simulink model "Control_test"  (R2014b)
settings: Solver=FixedStepDiscrete  StartTime=0.0  StopTime=Inf  FixedStep=0.001  RelTol=1e-3
PostLoadFcn:
  | , if any(exist('dsrtsu_mdlpostloadfcn', 'file') == [2, 3, 6]), try dsrtsu_mdlpostloadfcn('Execute', bdroot); catch fprintf('Error in PostLoadFcn (dsrtsu_mdlpostloadfcn) for model "%s":\n %s\n', bdroot, lasterr); end, end,
undefined symbols (not defined in the file or in its folder): dtLocal, slcm
libraries: rtican x163, simulink x14
(part 28 of 34)

== system Control_test/InputProcessing/RadarCanProcessing/Track54 ==
  Bus Creator : BusCreator  Inputs=12
  ESR_Track54 : rtican/RTICAN Receive (RX)   Reserved1=[]  Reserved2=[]  Reserved3=[]  Reserved4=[]  SfcnMessage=[]  Msg_Struct=[]  BoardTypeNo=[]  BoardNo=[]  ChannelNo=[]  Parameters=[]  DialogFcn=[]  UnitName=[]  Revision=[]  UnitValues=[]  DSProperties=struct('RTI',struct('Version',uint32(5),'BlockType',struct('isSLSource',uint8(1),'isSLSink',uint8(1),'isHWSource',uint8(0),'isHWSink',uint8(0),'isSetup',uint8(0),'isInline',uint8(1),'isNonInline',uint8(0),'isInterrupt',uint8(0),'isChannelwise',uint8(0)),'IOBoardType','RTICAN','UnitType','MESSAGE','Identifier','RX','DialogType','MSVC','BlockSet','RTICAN','SlaveProcessor','CAN'))  RTIBlockInterface=struct('OutputPortsWidth',int32([1 1 1 1 1 1 1 1 1 1 1 1]),'OutputPortsActive',[1 1 1 1 1 1 1 1 1 1 1 1],'OutputPortsName',{{'CAN_TX_TRACK_RANGE_RATE_54','CAN_TX_TRACK_MED_RANGE_MODE_54','CAN_TX_TRACK_RANGE_ACCEL_54','CAN_TX_TRACK_WIDTH_54','CAN_TX_TRACK_ROLLING_COUNT_54','CAN_TX_TRACK_BRIDGE_OBJECT_54','CAN_TX_TRACK_RANGE_54','CAN_TX_TRACK_ANGLE_54','CAN_TX_TRACK_STATUS_54','CAN_TX_TRACK_ONCOMING_54','CAN_TX_TRACK_GROUPING_CHANGED_54','CAN_TX_TRACK_LAT_RATE_54'}},'OutputPortsDataType',{{'SS_DOUBLE','SS_DOUBLE','SS_DOUBLE','SS_DOUBLE','SS_DOUBLE','SS_DOUBLE','SS_DOUBLE','SS_DOUBLE','SS_DOUBLE','SS_DOUBLE','SS_DOUBLE','SS_DOUBLE'}},'OutputPortsLabel',{{'CAN_TX_TRACK_RANGE_RATE_54','CAN_TX_TRACK_MED_RANGE_MODE_54','CAN_TX_TRACK_RANGE_ACCEL_54','CAN_TX_TRACK_WIDTH_54','CAN_TX_TRACK_ROLLING_COUNT_54','CAN_TX_TRACK_BRIDGE_OBJECT_54','CAN_TX_TRACK_RANGE_54','CAN_TX_TRACK_ANGLE_54','CAN_TX_TRACK_STATUS_54','CAN_TX_TRACK_ONCOMING_54','CAN_TX_TRACK_GROUPING_CHANGED_54','CAN_TX_TRACK_LAT_RATE_54'}},'OutputPortsLabelMode','ON','InputPortsWidth',int32(0),'InputPortsActive',0,'DialogFcn','rtican_message_interface_gui','BlockDisplay',{{'','center'}},'IconTransparency','on','ParameterTunableNames',{{}},'InitLevel',3,'BlockName',struct('Token',{{'ESR_Track54'}}),'SampleTime',{{0.01}},'TriggerPort',{{'none'}},'EnablePort',{{'none'}})  RTIBlockParameters=struct('BoardTypeNo',{{1,'OFF',[]}},'BoardNo',{{2,'ON',[1 16]}},'ChannelNo',{{2,'ON',[1 2]}},'Parameters',{{struct('DataFileSupport',struct('DataFileSelectedMaster',1,'DataFileSelectedLocal',0,'DataFileName','c:\users\mpc_car\documents\github\mpc-car\controller\dbcfiles\esr_dv3_64tgt.dbc|','DataFileDate',{{{['02-Nov-2012 20:32:52']},{['21-Mar-2013 13:39:53']},{['28-Sep-2011 17:08:52']}}},'SelectedFile',['<no file selected>'],'InterfaceFcn','rtican_dbc_file_parser'),'Options',struct('StatusSelected',0,'TimeSelected',0,'DeltaTimeSelected',0,'BytePortSelected',0,'MessageLengthSelected',0,'TriggerPort',struct('Selected',0,'TriggerType',0),'UserCoding',struct('Selected',0,'InterfaceFile','UserDecodingFile','FcnName','UserDecodeFcn','InportSelected',0,'InportWidth',1,'OutportSelected',0,'OutportWidth',1),'EnablePortSelected',0,'SignalOnPortnameSelected',1,'UseRXService',0),'Message',struct('MsgOnBlocknameSelected',1,'MsgName','ESR_Track54','MsgIdFormat',0,'MsgId',1333,'MsgLength',8,'NumSignals',12,'SampleTime',0.01,'Signal',struct('SgnName',{'CAN_TX_TRACK_RANGE_RATE_54','CAN_TX_TRACK_MED_RANGE_MODE_54','CAN_TX_TRACK_RANGE_ACCEL_54','CAN_TX_TRACK_WIDTH_54','CAN_TX_TRACK_ROLLING_COUNT_54','CAN_TX_TRACK_BRIDGE_OBJECT_54','CAN_TX_TRACK_RANGE_54','CAN_TX_TRACK_ANGLE_54','CAN_TX_TRACK_STATUS_54','CAN_TX_TRACK_ONCOMING_54','CAN_TX_TRACK_GROUPING_CHANGED_54','CAN_TX_TRACK_LAT_RATE_54'},'SgnStartBit',{0,14,16,26,30,31,32,43,53,56,57,58},'SgnLength',{14,2,10,4,1,1,11,10,3,1,1,6},'SgnType',{0,0,0,0,0,0,0,0,0,0,0,0},'ModeValue',{-1,-1,-1,-1,-1,-1,-1,-1,-1,-1,-1,-1},'DataType',{1,0,1,0,0,0,0,1,0,0,0,1},'ByteLayout',{2,2,2,2,2,2,2,2,2,2,2,2},'Factor',{0.01,1,0.05,0.5,1,1,0.1,0.1,1,1,1,0.25},'Offset',{0,0,0,0,0,0,0,0,0,0,0,0},'SgnComment',{{''},{''},{''},{''},{''},{''},{''},{''},{''},{''},{''},{''}},'SgnUnit',{'m/s','','m/s/s','m','','','m','deg','','','',''},'Min',{-81.92,0,-25.6,0,0,0,0,-51.2,0,0,0,-8},'Max',{81.91,3,25.55,7.5,1,0,204.7,51.1,7,0,0,7.75},'SLDataType',{'SS_DOUBLE','SS_DOUBLE','SS_DOUBLE','SS_DOUBLE','SS_DOUBLE','SS_DOUBLE','SS_DOUBLE','SS_DOUBLE','SS_DOUBLE','SS_DOUBLE','SS_DOUBLE','SS_DOUBLE'}),'MsgIdNumFormat',0,'MsgComment',{{''}}),'Version',1.2,'general',struct('isFromLib',0)),'OFF',[]}},'GroupId',{{struct('Group',{{'RTICAN'}},'No',4,'Behavior',{{'NAMECHANGE'}},'BlockType',{{'SINK'}},'NameChangeFlag',0),'OFF',[]}},'SFcnRTICANMessage',{{struct('MsgType','RX','SFcnPortType','Scalar','MsgName','ESR_Track54','MsgIdFormat','STD','MsgId',1333,'MsgLength',8,'NumSignals',12,'SampleTime',0.01,'Signal',struct('SgnName',{'CAN_TX_TRACK_RANGE_RATE_54','CAN_TX_TRACK_MED_RANGE_MODE_54','CAN_TX_TRACK_RANGE_ACCEL_54','CAN_TX_TRACK_WIDTH_54','CAN_TX_TRACK_ROLLING_COUNT_54','CAN_TX_TRACK_BRIDGE_OBJECT_54','CAN_TX_TRACK_RANGE_54','CAN_TX_TRACK_ANGLE_54','CAN_TX_TRACK_STATUS_54','CAN_TX_TRACK_ONCOMING_54','CAN_TX_TRACK_GROUPING_CHANGED_54','CAN_TX_TRACK_LAT_RATE_54'},'SgnStartBit',{0,14,16,26,30,31,32,43,53,56,57,58},'SgnLength',{14,2,10,4,1,1,11,10,3,1,1,6},'SgnType',{'standard','standard','standard','standard','standard','standard','standard','standard','standard','standard','standard','standard'},'ModeValue',{-1,-1,-1,-1,-1,-1,-1,-1,-1,-1,-1,-1},'DataType',{['signed int'],['unsigned int'],['signed int'],['unsigned int'],['unsigned int'],['unsigned int'],['unsigned int'],['signed int'],['unsigned int'],['unsigned int'],['unsigned int'],['signed int']},'ByteLayout',{['motorola back.'],['motorola back.'],['motorola back.'],['motorola back.'],['motorola back.'],['motorola back.'],['motorola back.'],['motorola back.'],['motorola back.'],['motorola back.'],['motorola back.'],['motorola back.']},'Factor',{0.01,1,0.05,0.5,1,1,0.1,0.1,1,1,1,0.25},'Offset',{0,0,0,0,0,0,0,0,0,0,0,0},'SLDataType',{'SS_DOUBLE','SS_DOUBLE','SS_DOUBLE','SS_DOUBLE','SS_DOUBLE','SS_DOUBLE','SS_DOUBLE','SS_DOUBLE','SS_DOUBLE','SS_DOUBLE','SS_DOUBLE','SS_DOUBLE'}),'StatusSelected','no','TimeSelected','no','DeltaTimeSelected','no','BytePortSelected','no','MessageLengthSelected','no','TriggerPort',struct('Selected','no','TriggerType',0),'UserCoding',struct('Selected','no','InterfaceFile','UserDecodingFile','FcnName','UserDecodeFcn','InportSelected','no','InportWidth',1,'OutportSelected','no','OutportWidth',1),'EnablePortSelected','no','UseRXService','no','BoardType','DS1','BoardNo',2,'ControllerNo',2),'OFF',[]}},'TLCFileName',{{'rtican_rx_message','OFF',[]}})  RTISFcnParameters=struct('SFcnRTICANMessage','struct','TLCFileName','char')  RTIBlockParaDefault=struct('BoardTypeNo',4302,'BoardNo',1,'ChannelNo',1,'Parameters',struct('DataFileSupport',struct('DataFileSelectedMaster',0,'DataFileSelectedLocal',0,'DataFileName','','DataFileDate','','SelectedFile',['<no file selected>']),'Options',struct('StatusSelected',1,'TimeSelected',1,'DeltaTimeSelected',1,'BytePortSelected',0,'MessageLengthSelected',0,'TriggerPort',struct('Selected',0,'TriggerType','rising'),'UserCoding',struct('Selected',0,'InterfaceFile','UserDecodingFile','FcnName','UserDecodeFcn','InportSelected',0,'InportWidth',1,'OutportSelected',0,'OutportWidth',1),'EnablePortSelected',0,'SignalOnPortnameSelected',1,'UseRXService',0),'Message',struct('MsgOnBlocknameSelected',0,'MsgName',['RX Message'],'MsgIdFormat',0,'MsgId',100,'MsgLength',8,'NumSignals',1,'SampleTime',-1,'Signal',struct('SgnName',['RX signal'],'SgnStartBit',0,'SgnLength',8,'SgnType',0,'ModeValue',-1,'DataType',0,'SLDataType','SS_DOUBLE','ByteLayout',0,'Factor',1,'Offset',0,'Min',0,'Max',255,'SgnComment',{{}},'SgnUnit',''),'MsgIdNumFormat',0,'MsgComment',{{''}}),'Version',1.2,'general',struct('isFromLib',1)),'GroupId',struct('Group',{{'RTICAN'}},'No',1,'Behavior',{{'NAMECHANGE'}},'BlockType',{{'SINK'}},'NameChangeFlag',0),'SFcnRTICANMessage',struct('MsgType','RX','MsgName',['RX Message'],'MsgIdFormat','STD','MsgId',100,'MsgLength',8,'NumSignals',1,'SampleTime',-1,'Signal',struct('SgnName',['RX signal'],'SgnStartBit',0,'SgnLength',8,'SgnType','standard','ModeValue',-1,'DataType',['unsigned int'],'ByteLayout',['little endian'],'SLDataType','SS_DOUBLE','Factor',1,'Offset',0),'StatusSelected','yes','TimeSelected','yes','DeltaTimeSelected','yes','BytePortSelected','no','MessageLengthSelected','no','EnablePortSelected','no','UserCoding',struct('Selected','no','InterfaceFile','UserDecodingFile','FcnName','UserDecodeFcn','InportSelected','no','InportWidth',1,'OutportSelected','no','OutportWidth',1),'TriggerPort',struct('Selected','no','TriggerType','rising'),'UseRXService','no','BoardType','DS4302','BoardNo',1,'ControllerNo',1,'SFcnPortType','Scalar'),'TLCFileName','rtican_rx_message')
      settings: AttributesFormatString=Group Id: RTICAN4\n
  Out1 : Outport
  wires:
  Bus Creator/1 -> Out1/1  "Track54"
  ESR_Track54/1 -> Bus Creator/1  "CAN_TX_TRACK_RANGE_RATE_54"
  ESR_Track54/2 -> Bus Creator/2  "CAN_TX_TRACK_MED_RANGE_MODE_54"
  ESR_Track54/3 -> Bus Creator/3  "CAN_TX_TRACK_RANGE_ACCEL_54"
  ESR_Track54/4 -> Bus Creator/4  "CAN_TX_TRACK_WIDTH_54"
  ESR_Track54/5 -> Bus Creator/5  "CAN_TX_TRACK_ROLLING_COUNT_54"
  ESR_Track54/6 -> Bus Creator/6  "CAN_TX_TRACK_BRIDGE_OBJECT_54"
  ESR_Track54/7 -> Bus Creator/7  "CAN_TX_TRACK_RANGE_54"
  ESR_Track54/8 -> Bus Creator/8  "CAN_TX_TRACK_ANGLE_54"
  ESR_Track54/9 -> Bus Creator/9  "CAN_TX_TRACK_STATUS_54"
  ESR_Track54/10 -> Bus Creator/10  "CAN_TX_TRACK_ONCOMING_54"
  ESR_Track54/11 -> Bus Creator/11  "CAN_TX_TRACK_GROUPING_CHANGED_54"
  ESR_Track54/12 -> Bus Creator/12  "CAN_TX_TRACK_LAT_RATE_54"

== system Control_test/InputProcessing/RadarCanProcessing/Track55 ==
  Bus Creator : BusCreator  Inputs=12
  ESR_Track55 : rtican/RTICAN Receive (RX)   Reserved1=[]  Reserved2=[]  Reserved3=[]  Reserved4=[]  SfcnMessage=[]  Msg_Struct=[]  BoardTypeNo=[]  BoardNo=[]  ChannelNo=[]  Parameters=[]  DialogFcn=[]  UnitName=[]  Revision=[]  UnitValues=[]  DSProperties=struct('RTI',struct('Version',uint32(5),'BlockType',struct('isSLSource',uint8(1),'isSLSink',uint8(1),'isHWSource',uint8(0),'isHWSink',uint8(0),'isSetup',uint8(0),'isInline',uint8(1),'isNonInline',uint8(0),'isInterrupt',uint8(0),'isChannelwise',uint8(0)),'IOBoardType','RTICAN','UnitType','MESSAGE','Identifier','RX','DialogType','MSVC','BlockSet','RTICAN','SlaveProcessor','CAN'))  RTIBlockInterface=struct('OutputPortsWidth',int32([1 1 1 1 1 1 1 1 1 1 1 1]),'OutputPortsActive',[1 1 1 1 1 1 1 1 1 1 1 1],'OutputPortsName',{{'CAN_TX_TRACK_RANGE_RATE_55','CAN_TX_TRACK_MED_RANGE_MODE_55','CAN_TX_TRACK_RANGE_ACCEL_55','CAN_TX_TRACK_WIDTH_55','CAN_TX_TRACK_ROLLING_COUNT_55','CAN_TX_TRACK_BRIDGE_OBJECT_55','CAN_TX_TRACK_RANGE_55','CAN_TX_TRACK_ANGLE_55','CAN_TX_TRACK_STATUS_55','CAN_TX_TRACK_ONCOMING_55','CAN_TX_TRACK_GROUPING_CHANGED_55','CAN_TX_TRACK_LAT_RATE_55'}},'OutputPortsDataType',{{'SS_DOUBLE','SS_DOUBLE','SS_DOUBLE','SS_DOUBLE','SS_DOUBLE','SS_DOUBLE','SS_DOUBLE','SS_DOUBLE','SS_DOUBLE','SS_DOUBLE','SS_DOUBLE','SS_DOUBLE'}},'OutputPortsLabel',{{'CAN_TX_TRACK_RANGE_RATE_55','CAN_TX_TRACK_MED_RANGE_MODE_55','CAN_TX_TRACK_RANGE_ACCEL_55','CAN_TX_TRACK_WIDTH_55','CAN_TX_TRACK_ROLLING_COUNT_55','CAN_TX_TRACK_BRIDGE_OBJECT_55','CAN_TX_TRACK_RANGE_55','CAN_TX_TRACK_ANGLE_55','CAN_TX_TRACK_STATUS_55','CAN_TX_TRACK_ONCOMING_55','CAN_TX_TRACK_GROUPING_CHANGED_55','CAN_TX_TRACK_LAT_RATE_55'}},'OutputPortsLabelMode','ON','InputPortsWidth',int32(0),'InputPortsActive',0,'DialogFcn','rtican_message_interface_gui','BlockDisplay',{{'','center'}},'IconTransparency','on','ParameterTunableNames',{{}},'InitLevel',3,'BlockName',struct('Token',{{'ESR_Track55'}}),'SampleTime',{{0.01}},'TriggerPort',{{'none'}},'EnablePort',{{'none'}})  RTIBlockParameters=struct('BoardTypeNo',{{1,'OFF',[]}},'BoardNo',{{2,'ON',[1 16]}},'ChannelNo',{{2,'ON',[1 2]}},'Parameters',{{struct('DataFileSupport',struct('DataFileSelectedMaster',1,'DataFileSelectedLocal',0,'DataFileName','c:\users\mpc_car\documents\github\mpc-car\controller\dbcfiles\esr_dv3_64tgt.dbc|','DataFileDate',{{{['02-Nov-2012 20:32:52']},{['21-Mar-2013 13:39:53']},{['28-Sep-2011 17:08:52']}}},'SelectedFile',['<no file selected>'],'InterfaceFcn','rtican_dbc_file_parser'),'Options',struct('StatusSelected',0,'TimeSelected',0,'DeltaTimeSelected',0,'BytePortSelected',0,'MessageLengthSelected',0,'TriggerPort',struct('Selected',0,'TriggerType',0),'UserCoding',struct('Selected',0,'InterfaceFile','UserDecodingFile','FcnName','UserDecodeFcn','InportSelected',0,'InportWidth',1,'OutportSelected',0,'OutportWidth',1),'EnablePortSelected',0,'SignalOnPortnameSelected',1,'UseRXService',0),'Message',struct('MsgOnBlocknameSelected',1,'MsgName','ESR_Track55','MsgIdFormat',0,'MsgId',1334,'MsgLength',8,'NumSignals',12,'SampleTime',0.01,'Signal',struct('SgnName',{'CAN_TX_TRACK_RANGE_RATE_55','CAN_TX_TRACK_MED_RANGE_MODE_55','CAN_TX_TRACK_RANGE_ACCEL_55','CAN_TX_TRACK_WIDTH_55','CAN_TX_TRACK_ROLLING_COUNT_55','CAN_TX_TRACK_BRIDGE_OBJECT_55','CAN_TX_TRACK_RANGE_55','CAN_TX_TRACK_ANGLE_55','CAN_TX_TRACK_STATUS_55','CAN_TX_TRACK_ONCOMING_55','CAN_TX_TRACK_GROUPING_CHANGED_55','CAN_TX_TRACK_LAT_RATE_55'},'SgnStartBit',{0,14,16,26,30,31,32,43,53,56,57,58},'SgnLength',{14,2,10,4,1,1,11,10,3,1,1,6},'SgnType',{0,0,0,0,0,0,0,0,0,0,0,0},'ModeValue',{-1,-1,-1,-1,-1,-1,-1,-1,-1,-1,-1,-1},'DataType',{1,0,1,0,0,0,0,1,0,0,0,1},'ByteLayout',{2,2,2,2,2,2,2,2,2,2,2,2},'Factor',{0.01,1,0.05,0.5,1,1,0.1,0.1,1,1,1,0.25},'Offset',{0,0,0,0,0,0,0,0,0,0,0,0},'SgnComment',{{''},{''},{''},{''},{''},{''},{''},{''},{''},{''},{''},{''}},'SgnUnit',{'m/s','','m/s/s','m','','','m','deg','','','',''},'Min',{-81.92,0,-25.6,0,0,0,0,-51.2,0,0,0,-8},'Max',{81.91,3,25.55,7.5,1,0,204.7,51.1,7,0,0,7.75},'SLDataType',{'SS_DOUBLE','SS_DOUBLE','SS_DOUBLE','SS_DOUBLE','SS_DOUBLE','SS_DOUBLE','SS_DOUBLE','SS_DOUBLE','SS_DOUBLE','SS_DOUBLE','SS_DOUBLE','SS_DOUBLE'}),'MsgIdNumFormat',0,'MsgComment',{{''}}),'Version',1.2,'general',struct('isFromLib',0)),'OFF',[]}},'GroupId',{{struct('Group',{{'RTICAN'}},'No',4,'Behavior',{{'NAMECHANGE'}},'BlockType',{{'SINK'}},'NameChangeFlag',0),'OFF',[]}},'SFcnRTICANMessage',{{struct('MsgType','RX','SFcnPortType','Scalar','MsgName','ESR_Track55','MsgIdFormat','STD','MsgId',1334,'MsgLength',8,'NumSignals',12,'SampleTime',0.01,'Signal',struct('SgnName',{'CAN_TX_TRACK_RANGE_RATE_55','CAN_TX_TRACK_MED_RANGE_MODE_55','CAN_TX_TRACK_RANGE_ACCEL_55','CAN_TX_TRACK_WIDTH_55','CAN_TX_TRACK_ROLLING_COUNT_55','CAN_TX_TRACK_BRIDGE_OBJECT_55','CAN_TX_TRACK_RANGE_55','CAN_TX_TRACK_ANGLE_55','CAN_TX_TRACK_STATUS_55','CAN_TX_TRACK_ONCOMING_55','CAN_TX_TRACK_GROUPING_CHANGED_55','CAN_TX_TRACK_LAT_RATE_55'},'SgnStartBit',{0,14,16,26,30,31,32,43,53,56,57,58},'SgnLength',{14,2,10,4,1,1,11,10,3,1,1,6},'SgnType',{'standard','standard','standard','standard','standard','standard','standard','standard','standard','standard','standard','standard'},'ModeValue',{-1,-1,-1,-1,-1,-1,-1,-1,-1,-1,-1,-1},'DataType',{['signed int'],['unsigned int'],['signed int'],['unsigned int'],['unsigned int'],['unsigned int'],['unsigned int'],['signed int'],['unsigned int'],['unsigned int'],['unsigned int'],['signed int']},'ByteLayout',{['motorola back.'],['motorola back.'],['motorola back.'],['motorola back.'],['motorola back.'],['motorola back.'],['motorola back.'],['motorola back.'],['motorola back.'],['motorola back.'],['motorola back.'],['motorola back.']},'Factor',{0.01,1,0.05,0.5,1,1,0.1,0.1,1,1,1,0.25},'Offset',{0,0,0,0,0,0,0,0,0,0,0,0},'SLDataType',{'SS_DOUBLE','SS_DOUBLE','SS_DOUBLE','SS_DOUBLE','SS_DOUBLE','SS_DOUBLE','SS_DOUBLE','SS_DOUBLE','SS_DOUBLE','SS_DOUBLE','SS_DOUBLE','SS_DOUBLE'}),'StatusSelected','no','TimeSelected','no','DeltaTimeSelected','no','BytePortSelected','no','MessageLengthSelected','no','TriggerPort',struct('Selected','no','TriggerType',0),'UserCoding',struct('Selected','no','InterfaceFile','UserDecodingFile','FcnName','UserDecodeFcn','InportSelected','no','InportWidth',1,'OutportSelected','no','OutportWidth',1),'EnablePortSelected','no','UseRXService','no','BoardType','DS1','BoardNo',2,'ControllerNo',2),'OFF',[]}},'TLCFileName',{{'rtican_rx_message','OFF',[]}})  RTISFcnParameters=struct('SFcnRTICANMessage','struct','TLCFileName','char')  RTIBlockParaDefault=struct('BoardTypeNo',4302,'BoardNo',1,'ChannelNo',1,'Parameters',struct('DataFileSupport',struct('DataFileSelectedMaster',0,'DataFileSelectedLocal',0,'DataFileName','','DataFileDate','','SelectedFile',['<no file selected>']),'Options',struct('StatusSelected',1,'TimeSelected',1,'DeltaTimeSelected',1,'BytePortSelected',0,'MessageLengthSelected',0,'TriggerPort',struct('Selected',0,'TriggerType','rising'),'UserCoding',struct('Selected',0,'InterfaceFile','UserDecodingFile','FcnName','UserDecodeFcn','InportSelected',0,'InportWidth',1,'OutportSelected',0,'OutportWidth',1),'EnablePortSelected',0,'SignalOnPortnameSelected',1,'UseRXService',0),'Message',struct('MsgOnBlocknameSelected',0,'MsgName',['RX Message'],'MsgIdFormat',0,'MsgId',100,'MsgLength',8,'NumSignals',1,'SampleTime',-1,'Signal',struct('SgnName',['RX signal'],'SgnStartBit',0,'SgnLength',8,'SgnType',0,'ModeValue',-1,'DataType',0,'SLDataType','SS_DOUBLE','ByteLayout',0,'Factor',1,'Offset',0,'Min',0,'Max',255,'SgnComment',{{}},'SgnUnit',''),'MsgIdNumFormat',0,'MsgComment',{{''}}),'Version',1.2,'general',struct('isFromLib',1)),'GroupId',struct('Group',{{'RTICAN'}},'No',1,'Behavior',{{'NAMECHANGE'}},'BlockType',{{'SINK'}},'NameChangeFlag',0),'SFcnRTICANMessage',struct('MsgType','RX','MsgName',['RX Message'],'MsgIdFormat','STD','MsgId',100,'MsgLength',8,'NumSignals',1,'SampleTime',-1,'Signal',struct('SgnName',['RX signal'],'SgnStartBit',0,'SgnLength',8,'SgnType','standard','ModeValue',-1,'DataType',['unsigned int'],'ByteLayout',['little endian'],'SLDataType','SS_DOUBLE','Factor',1,'Offset',0),'StatusSelected','yes','TimeSelected','yes','DeltaTimeSelected','yes','BytePortSelected','no','MessageLengthSelected','no','EnablePortSelected','no','UserCoding',struct('Selected','no','InterfaceFile','UserDecodingFile','FcnName','UserDecodeFcn','InportSelected','no','InportWidth',1,'OutportSelected','no','OutportWidth',1),'TriggerPort',struct('Selected','no','TriggerType','rising'),'UseRXService','no','BoardType','DS4302','BoardNo',1,'ControllerNo',1,'SFcnPortType','Scalar'),'TLCFileName','rtican_rx_message')
      settings: AttributesFormatString=Group Id: RTICAN4\n
  Out1 : Outport
  wires:
  Bus Creator/1 -> Out1/1  "Track55"
  ESR_Track55/1 -> Bus Creator/1  "CAN_TX_TRACK_RANGE_RATE_55"
  ESR_Track55/2 -> Bus Creator/2  "CAN_TX_TRACK_MED_RANGE_MODE_55"
  ESR_Track55/3 -> Bus Creator/3  "CAN_TX_TRACK_RANGE_ACCEL_55"
  ESR_Track55/4 -> Bus Creator/4  "CAN_TX_TRACK_WIDTH_55"
  ESR_Track55/5 -> Bus Creator/5  "CAN_TX_TRACK_ROLLING_COUNT_55"
  ESR_Track55/6 -> Bus Creator/6  "CAN_TX_TRACK_BRIDGE_OBJECT_55"
  ESR_Track55/7 -> Bus Creator/7  "CAN_TX_TRACK_RANGE_55"
  ESR_Track55/8 -> Bus Creator/8  "CAN_TX_TRACK_ANGLE_55"
  ESR_Track55/9 -> Bus Creator/9  "CAN_TX_TRACK_STATUS_55"
  ESR_Track55/10 -> Bus Creator/10  "CAN_TX_TRACK_ONCOMING_55"
  ESR_Track55/11 -> Bus Creator/11  "CAN_TX_TRACK_GROUPING_CHANGED_55"
  ESR_Track55/12 -> Bus Creator/12  "CAN_TX_TRACK_LAT_RATE_55"

== system Control_test/InputProcessing/RadarCanProcessing/Track56 ==
  Bus Creator : BusCreator  Inputs=12
  ESR_Track56 : rtican/RTICAN Receive (RX)   Reserved1=[]  Reserved2=[]  Reserved3=[]  Reserved4=[]  SfcnMessage=[]  Msg_Struct=[]  BoardTypeNo=[]  BoardNo=[]  ChannelNo=[]  Parameters=[]  DialogFcn=[]  UnitName=[]  Revision=[]  UnitValues=[]  DSProperties=struct('RTI',struct('Version',uint32(5),'BlockType',struct('isSLSource',uint8(1),'isSLSink',uint8(1),'isHWSource',uint8(0),'isHWSink',uint8(0),'isSetup',uint8(0),'isInline',uint8(1),'isNonInline',uint8(0),'isInterrupt',uint8(0),'isChannelwise',uint8(0)),'IOBoardType','RTICAN','UnitType','MESSAGE','Identifier','RX','DialogType','MSVC','BlockSet','RTICAN','SlaveProcessor','CAN'))  RTIBlockInterface=struct('OutputPortsWidth',int32([1 1 1 1 1 1 1 1 1 1 1 1]),'OutputPortsActive',[1 1 1 1 1 1 1 1 1 1 1 1],'OutputPortsName',{{'CAN_TX_TRACK_RANGE_RATE_56','CAN_TX_TRACK_MED_RANGE_MODE_56','CAN_TX_TRACK_RANGE_ACCEL_56','CAN_TX_TRACK_WIDTH_56','CAN_TX_TRACK_ROLLING_COUNT_56','CAN_TX_TRACK_BRIDGE_OBJECT_56','CAN_TX_TRACK_RANGE_56','CAN_TX_TRACK_ANGLE_56','CAN_TX_TRACK_STATUS_56','CAN_TX_TRACK_ONCOMING_56','CAN_TX_TRACK_GROUPING_CHANGED_56','CAN_TX_TRACK_LAT_RATE_56'}},'OutputPortsDataType',{{'SS_DOUBLE','SS_DOUBLE','SS_DOUBLE','SS_DOUBLE','SS_DOUBLE','SS_DOUBLE','SS_DOUBLE','SS_DOUBLE','SS_DOUBLE','SS_DOUBLE','SS_DOUBLE','SS_DOUBLE'}},'OutputPortsLabel',{{'CAN_TX_TRACK_RANGE_RATE_56','CAN_TX_TRACK_MED_RANGE_MODE_56','CAN_TX_TRACK_RANGE_ACCEL_56','CAN_TX_TRACK_WIDTH_56','CAN_TX_TRACK_ROLLING_COUNT_56','CAN_TX_TRACK_BRIDGE_OBJECT_56','CAN_TX_TRACK_RANGE_56','CAN_TX_TRACK_ANGLE_56','CAN_TX_TRACK_STATUS_56','CAN_TX_TRACK_ONCOMING_56','CAN_TX_TRACK_GROUPING_CHANGED_56','CAN_TX_TRACK_LAT_RATE_56'}},'OutputPortsLabelMode','ON','InputPortsWidth',int32(0),'InputPortsActive',0,'DialogFcn','rtican_message_interface_gui','BlockDisplay',{{'','center'}},'IconTransparency','on','ParameterTunableNames',{{}},'InitLevel',3,'BlockName',struct('Token',{{'ESR_Track56'}}),'SampleTime',{{0.01}},'TriggerPort',{{'none'}},'EnablePort',{{'none'}})  RTIBlockParameters=struct('BoardTypeNo',{{1,'OFF',[]}},'BoardNo',{{2,'ON',[1 16]}},'ChannelNo',{{2,'ON',[1 2]}},'Parameters',{{struct('DataFileSupport',struct('DataFileSelectedMaster',1,'DataFileSelectedLocal',0,'DataFileName','c:\users\mpc_car\documents\github\mpc-car\controller\dbcfiles\esr_dv3_64tgt.dbc|','DataFileDate',{{{['02-Nov-2012 20:32:52']},{['21-Mar-2013 13:39:53']},{['28-Sep-2011 17:08:52']}}},'SelectedFile',['<no file selected>'],'InterfaceFcn','rtican_dbc_file_parser'),'Options',struct('StatusSelected',0,'TimeSelected',0,'DeltaTimeSelected',0,'BytePortSelected',0,'MessageLengthSelected',0,'TriggerPort',struct('Selected',0,'TriggerType',0),'UserCoding',struct('Selected',0,'InterfaceFile','UserDecodingFile','FcnName','UserDecodeFcn','InportSelected',0,'InportWidth',1,'OutportSelected',0,'OutportWidth',1),'EnablePortSelected',0,'SignalOnPortnameSelected',1,'UseRXService',0),'Message',struct('MsgOnBlocknameSelected',1,'MsgName','ESR_Track56','MsgIdFormat',0,'MsgId',1335,'MsgLength',8,'NumSignals',12,'SampleTime',0.01,'Signal',struct('SgnName',{'CAN_TX_TRACK_RANGE_RATE_56','CAN_TX_TRACK_MED_RANGE_MODE_56','CAN_TX_TRACK_RANGE_ACCEL_56','CAN_TX_TRACK_WIDTH_56','CAN_TX_TRACK_ROLLING_COUNT_56','CAN_TX_TRACK_BRIDGE_OBJECT_56','CAN_TX_TRACK_RANGE_56','CAN_TX_TRACK_ANGLE_56','CAN_TX_TRACK_STATUS_56','CAN_TX_TRACK_ONCOMING_56','CAN_TX_TRACK_GROUPING_CHANGED_56','CAN_TX_TRACK_LAT_RATE_56'},'SgnStartBit',{0,14,16,26,30,31,32,43,53,56,57,58},'SgnLength',{14,2,10,4,1,1,11,10,3,1,1,6},'SgnType',{0,0,0,0,0,0,0,0,0,0,0,0},'ModeValue',{-1,-1,-1,-1,-1,-1,-1,-1,-1,-1,-1,-1},'DataType',{1,0,1,0,0,0,0,1,0,0,0,1},'ByteLayout',{2,2,2,2,2,2,2,2,2,2,2,2},'Factor',{0.01,1,0.05,0.5,1,1,0.1,0.1,1,1,1,0.25},'Offset',{0,0,0,0,0,0,0,0,0,0,0,0},'SgnComment',{{''},{''},{''},{''},{''},{''},{''},{''},{''},{''},{''},{''}},'SgnUnit',{'m/s','','m/s/s','m','','','m','deg','','','',''},'Min',{-81.92,0,-25.6,0,0,0,0,-51.2,0,0,0,-8},'Max',{81.91,3,25.55,7.5,1,0,204.7,51.1,7,0,0,7.75},'SLDataType',{'SS_DOUBLE','SS_DOUBLE','SS_DOUBLE','SS_DOUBLE','SS_DOUBLE','SS_DOUBLE','SS_DOUBLE','SS_DOUBLE','SS_DOUBLE','SS_DOUBLE','SS_DOUBLE','SS_DOUBLE'}),'MsgIdNumFormat',0,'MsgComment',{{''}}),'Version',1.2,'general',struct('isFromLib',0)),'OFF',[]}},'GroupId',{{struct('Group',{{'RTICAN'}},'No',4,'Behavior',{{'NAMECHANGE'}},'BlockType',{{'SINK'}},'NameChangeFlag',0),'OFF',[]}},'SFcnRTICANMessage',{{struct('MsgType','RX','SFcnPortType','Scalar','MsgName','ESR_Track56','MsgIdFormat','STD','MsgId',1335,'MsgLength',8,'NumSignals',12,'SampleTime',0.01,'Signal',struct('SgnName',{'CAN_TX_TRACK_RANGE_RATE_56','CAN_TX_TRACK_MED_RANGE_MODE_56','CAN_TX_TRACK_RANGE_ACCEL_56','CAN_TX_TRACK_WIDTH_56','CAN_TX_TRACK_ROLLING_COUNT_56','CAN_TX_TRACK_BRIDGE_OBJECT_56','CAN_TX_TRACK_RANGE_56','CAN_TX_TRACK_ANGLE_56','CAN_TX_TRACK_STATUS_56','CAN_TX_TRACK_ONCOMING_56','CAN_TX_TRACK_GROUPING_CHANGED_56','CAN_TX_TRACK_LAT_RATE_56'},'SgnStartBit',{0,14,16,26,30,31,32,43,53,56,57,58},'SgnLength',{14,2,10,4,1,1,11,10,3,1,1,6},'SgnType',{'standard','standard','standard','standard','standard','standard','standard','standard','standard','standard','standard','standard'},'ModeValue',{-1,-1,-1,-1,-1,-1,-1,-1,-1,-1,-1,-1},'DataType',{['signed int'],['unsigned int'],['signed int'],['unsigned int'],['unsigned int'],['unsigned int'],['unsigned int'],['signed int'],['unsigned int'],['unsigned int'],['unsigned int'],['signed int']},'ByteLayout',{['motorola back.'],['motorola back.'],['motorola back.'],['motorola back.'],['motorola back.'],['motorola back.'],['motorola back.'],['motorola back.'],['motorola back.'],['motorola back.'],['motorola back.'],['motorola back.']},'Factor',{0.01,1,0.05,0.5,1,1,0.1,0.1,1,1,1,0.25},'Offset',{0,0,0,0,0,0,0,0,0,0,0,0},'SLDataType',{'SS_DOUBLE','SS_DOUBLE','SS_DOUBLE','SS_DOUBLE','SS_DOUBLE','SS_DOUBLE','SS_DOUBLE','SS_DOUBLE','SS_DOUBLE','SS_DOUBLE','SS_DOUBLE','SS_DOUBLE'}),'StatusSelected','no','TimeSelected','no','DeltaTimeSelected','no','BytePortSelected','no','MessageLengthSelected','no','TriggerPort',struct('Selected','no','TriggerType',0),'UserCoding',struct('Selected','no','InterfaceFile','UserDecodingFile','FcnName','UserDecodeFcn','InportSelected','no','InportWidth',1,'OutportSelected','no','OutportWidth',1),'EnablePortSelected','no','UseRXService','no','BoardType','DS1','BoardNo',2,'ControllerNo',2),'OFF',[]}},'TLCFileName',{{'rtican_rx_message','OFF',[]}})  RTISFcnParameters=struct('SFcnRTICANMessage','struct','TLCFileName','char')  RTIBlockParaDefault=struct('BoardTypeNo',4302,'BoardNo',1,'ChannelNo',1,'Parameters',struct('DataFileSupport',struct('DataFileSelectedMaster',0,'DataFileSelectedLocal',0,'DataFileName','','DataFileDate','','SelectedFile',['<no file selected>']),'Options',struct('StatusSelected',1,'TimeSelected',1,'DeltaTimeSelected',1,'BytePortSelected',0,'MessageLengthSelected',0,'TriggerPort',struct('Selected',0,'TriggerType','rising'),'UserCoding',struct('Selected',0,'InterfaceFile','UserDecodingFile','FcnName','UserDecodeFcn','InportSelected',0,'InportWidth',1,'OutportSelected',0,'OutportWidth',1),'EnablePortSelected',0,'SignalOnPortnameSelected',1,'UseRXService',0),'Message',struct('MsgOnBlocknameSelected',0,'MsgName',['RX Message'],'MsgIdFormat',0,'MsgId',100,'MsgLength',8,'NumSignals',1,'SampleTime',-1,'Signal',struct('SgnName',['RX signal'],'SgnStartBit',0,'SgnLength',8,'SgnType',0,'ModeValue',-1,'DataType',0,'SLDataType','SS_DOUBLE','ByteLayout',0,'Factor',1,'Offset',0,'Min',0,'Max',255,'SgnComment',{{}},'SgnUnit',''),'MsgIdNumFormat',0,'MsgComment',{{''}}),'Version',1.2,'general',struct('isFromLib',1)),'GroupId',struct('Group',{{'RTICAN'}},'No',1,'Behavior',{{'NAMECHANGE'}},'BlockType',{{'SINK'}},'NameChangeFlag',0),'SFcnRTICANMessage',struct('MsgType','RX','MsgName',['RX Message'],'MsgIdFormat','STD','MsgId',100,'MsgLength',8,'NumSignals',1,'SampleTime',-1,'Signal',struct('SgnName',['RX signal'],'SgnStartBit',0,'SgnLength',8,'SgnType','standard','ModeValue',-1,'DataType',['unsigned int'],'ByteLayout',['little endian'],'SLDataType','SS_DOUBLE','Factor',1,'Offset',0),'StatusSelected','yes','TimeSelected','yes','DeltaTimeSelected','yes','BytePortSelected','no','MessageLengthSelected','no','EnablePortSelected','no','UserCoding',struct('Selected','no','InterfaceFile','UserDecodingFile','FcnName','UserDecodeFcn','InportSelected','no','InportWidth',1,'OutportSelected','no','OutportWidth',1),'TriggerPort',struct('Selected','no','TriggerType','rising'),'UseRXService','no','BoardType','DS4302','BoardNo',1,'ControllerNo',1,'SFcnPortType','Scalar'),'TLCFileName','rtican_rx_message')
      settings: AttributesFormatString=Group Id: RTICAN4\n
  Out1 : Outport
  wires:
  Bus Creator/1 -> Out1/1  "Track56"
  ESR_Track56/1 -> Bus Creator/1  "CAN_TX_TRACK_RANGE_RATE_56"
  ESR_Track56/2 -> Bus Creator/2  "CAN_TX_TRACK_MED_RANGE_MODE_56"
  ESR_Track56/3 -> Bus Creator/3  "CAN_TX_TRACK_RANGE_ACCEL_56"
  ESR_Track56/4 -> Bus Creator/4  "CAN_TX_TRACK_WIDTH_56"
  ESR_Track56/5 -> Bus Creator/5  "CAN_TX_TRACK_ROLLING_COUNT_56"
  ESR_Track56/6 -> Bus Creator/6  "CAN_TX_TRACK_BRIDGE_OBJECT_56"
  ESR_Track56/7 -> Bus Creator/7  "CAN_TX_TRACK_RANGE_56"
  ESR_Track56/8 -> Bus Creator/8  "CAN_TX_TRACK_ANGLE_56"
  ESR_Track56/9 -> Bus Creator/9  "CAN_TX_TRACK_STATUS_56"
  ESR_Track56/10 -> Bus Creator/10  "CAN_TX_TRACK_ONCOMING_56"
  ESR_Track56/11 -> Bus Creator/11  "CAN_TX_TRACK_GROUPING_CHANGED_56"
  ESR_Track56/12 -> Bus Creator/12  "CAN_TX_TRACK_LAT_RATE_56"

== system Control_test/InputProcessing/RadarCanProcessing/Track57 ==
  Bus Creator : BusCreator  Inputs=12
  ESR_Track57 : rtican/RTICAN Receive (RX)   Reserved1=[]  Reserved2=[]  Reserved3=[]  Reserved4=[]  SfcnMessage=[]  Msg_Struct=[]  BoardTypeNo=[]  BoardNo=[]  ChannelNo=[]  Parameters=[]  DialogFcn=[]  UnitName=[]  Revision=[]  UnitValues=[]  DSProperties=struct('RTI',struct('Version',uint32(5),'BlockType',struct('isSLSource',uint8(1),'isSLSink',uint8(1),'isHWSource',uint8(0),'isHWSink',uint8(0),'isSetup',uint8(0),'isInline',uint8(1),'isNonInline',uint8(0),'isInterrupt',uint8(0),'isChannelwise',uint8(0)),'IOBoardType','RTICAN','UnitType','MESSAGE','Identifier','RX','DialogType','MSVC','BlockSet','RTICAN','SlaveProcessor','CAN'))  RTIBlockInterface=struct('OutputPortsWidth',int32([1 1 1 1 1 1 1 1 1 1 1 1]),'OutputPortsActive',[1 1 1 1 1 1 1 1 1 1 1 1],'OutputPortsName',{{'CAN_TX_TRACK_RANGE_RATE_57','CAN_TX_TRACK_MED_RANGE_MODE_57','CAN_TX_TRACK_RANGE_ACCEL_57','CAN_TX_TRACK_WIDTH_57','CAN_TX_TRACK_ROLLING_COUNT_57','CAN_TX_TRACK_BRIDGE_OBJECT_57','CAN_TX_TRACK_RANGE_57','CAN_TX_TRACK_ANGLE_57','CAN_TX_TRACK_STATUS_57','CAN_TX_TRACK_ONCOMING_57','CAN_TX_TRACK_GROUPING_CHANGED_57','CAN_TX_TRACK_LAT_RATE_57'}},'OutputPortsDataType',{{'SS_DOUBLE','SS_DOUBLE','SS_DOUBLE','SS_DOUBLE','SS_DOUBLE','SS_DOUBLE','SS_DOUBLE','SS_DOUBLE','SS_DOUBLE','SS_DOUBLE','SS_DOUBLE','SS_DOUBLE'}},'OutputPortsLabel',{{'CAN_TX_TRACK_RANGE_RATE_57','CAN_TX_TRACK_MED_RANGE_MODE_57','CAN_TX_TRACK_RANGE_ACCEL_57','CAN_TX_TRACK_WIDTH_57','CAN_TX_TRACK_ROLLING_COUNT_57','CAN_TX_TRACK_BRIDGE_OBJECT_57','CAN_TX_TRACK_RANGE_57','CAN_TX_TRACK_ANGLE_57','CAN_TX_TRACK_STATUS_57','CAN_TX_TRACK_ONCOMING_57','CAN_TX_TRACK_GROUPING_CHANGED_57','CAN_TX_TRACK_LAT_RATE_57'}},'OutputPortsLabelMode','ON','InputPortsWidth',int32(0),'InputPortsActive',0,'DialogFcn','rtican_message_interface_gui','BlockDisplay',{{'','center'}},'IconTransparency','on','ParameterTunableNames',{{}},'InitLevel',3,'BlockName',struct('Token',{{'ESR_Track57'}}),'SampleTime',{{0.01}},'TriggerPort',{{'none'}},'EnablePort',{{'none'}})  RTIBlockParameters=struct('BoardTypeNo',{{1,'OFF',[]}},'BoardNo',{{2,'ON',[1 16]}},'ChannelNo',{{2,'ON',[1 2]}},'Parameters',{{struct('DataFileSupport',struct('DataFileSelectedMaster',1,'DataFileSelectedLocal',0,'DataFileName','c:\users\mpc_car\documents\github\mpc-car\controller\dbcfiles\esr_dv3_64tgt.dbc|','DataFileDate',{{{['02-Nov-2012 20:32:52']},{['21-Mar-2013 13:39:53']},{['28-Sep-2011 17:08:52']}}},'SelectedFile',['<no file selected>'],'InterfaceFcn','rtican_dbc_file_parser'),'Options',struct('StatusSelected',0,'TimeSelected',0,'DeltaTimeSelected',0,'BytePortSelected',0,'MessageLengthSelected',0,'TriggerPort',struct('Selected',0,'TriggerType',0),'UserCoding',struct('Selected',0,'InterfaceFile','UserDecodingFile','FcnName','UserDecodeFcn','InportSelected',0,'InportWidth',1,'OutportSelected',0,'OutportWidth',1),'EnablePortSelected',0,'SignalOnPortnameSelected',1,'UseRXService',0),'Message',struct('MsgOnBlocknameSelected',1,'MsgName','ESR_Track57','MsgIdFormat',0,'MsgId',1336,'MsgLength',8,'NumSignals',12,'SampleTime',0.01,'Signal',struct('SgnName',{'CAN_TX_TRACK_RANGE_RATE_57','CAN_TX_TRACK_MED_RANGE_MODE_57','CAN_TX_TRACK_RANGE_ACCEL_57','CAN_TX_TRACK_WIDTH_57','CAN_TX_TRACK_ROLLING_COUNT_57','CAN_TX_TRACK_BRIDGE_OBJECT_57','CAN_TX_TRACK_RANGE_57','CAN_TX_TRACK_ANGLE_57','CAN_TX_TRACK_STATUS_57','CAN_TX_TRACK_ONCOMING_57','CAN_TX_TRACK_GROUPING_CHANGED_57','CAN_TX_TRACK_LAT_RATE_57'},'SgnStartBit',{0,14,16,26,30,31,32,43,53,56,57,58},'SgnLength',{14,2,10,4,1,1,11,10,3,1,1,6},'SgnType',{0,0,0,0,0,0,0,0,0,0,0,0},'ModeValue',{-1,-1,-1,-1,-1,-1,-1,-1,-1,-1,-1,-1},'DataType',{1,0,1,0,0,0,0,1,0,0,0,1},'ByteLayout',{2,2,2,2,2,2,2,2,2,2,2,2},'Factor',{0.01,1,0.05,0.5,1,1,0.1,0.1,1,1,1,0.25},'Offset',{0,0,0,0,0,0,0,0,0,0,0,0},'SgnComment',{{''},{''},{''},{''},{''},{''},{''},{''},{''},{''},{''},{''}},'SgnUnit',{'m/s','','m/s/s','m','','','m','deg','','','',''},'Min',{-81.92,0,-25.6,0,0,0,0,-51.2,0,0,0,-8},'Max',{81.91,3,25.55,7.5,1,0,204.7,51.1,7,0,0,7.75},'SLDataType',{'SS_DOUBLE','SS_DOUBLE','SS_DOUBLE','SS_DOUBLE','SS_DOUBLE','SS_DOUBLE','SS_DOUBLE','SS_DOUBLE','SS_DOUBLE','SS_DOUBLE','SS_DOUBLE','SS_DOUBLE'}),'MsgIdNumFormat',0,'MsgComment',{{''}}),'Version',1.2,'general',struct('isFromLib',0)),'OFF',[]}},'GroupId',{{struct('Group',{{'RTICAN'}},'No',4,'Behavior',{{'NAMECHANGE'}},'BlockType',{{'SINK'}},'NameChangeFlag',0),'OFF',[]}},'SFcnRTICANMessage',{{struct('MsgType','RX','SFcnPortType','Scalar','MsgName','ESR_Track57','MsgIdFormat','STD','MsgId',1336,'MsgLength',8,'NumSignals',12,'SampleTime',0.01,'Signal',struct('SgnName',{'CAN_TX_TRACK_RANGE_RATE_57','CAN_TX_TRACK_MED_RANGE_MODE_57','CAN_TX_TRACK_RANGE_ACCEL_57','CAN_TX_TRACK_WIDTH_57','CAN_TX_TRACK_ROLLING_COUNT_57','CAN_TX_TRACK_BRIDGE_OBJECT_57','CAN_TX_TRACK_RANGE_57','CAN_TX_TRACK_ANGLE_57','CAN_TX_TRACK_STATUS_57','CAN_TX_TRACK_ONCOMING_57','CAN_TX_TRACK_GROUPING_CHANGED_57','CAN_TX_TRACK_LAT_RATE_57'},'SgnStartBit',{0,14,16,26,30,31,32,43,53,56,57,58},'SgnLength',{14,2,10,4,1,1,11,10,3,1,1,6},'SgnType',{'standard','standard','standard','standard','standard','standard','standard','standard','standard','standard','standard','standard'},'ModeValue',{-1,-1,-1,-1,-1,-1,-1,-1,-1,-1,-1,-1},'DataType',{['signed int'],['unsigned int'],['signed int'],['unsigned int'],['unsigned int'],['unsigned int'],['unsigned int'],['signed int'],['unsigned int'],['unsigned int'],['unsigned int'],['signed int']},'ByteLayout',{['motorola back.'],['motorola back.'],['motorola back.'],['motorola back.'],['motorola back.'],['motorola back.'],['motorola back.'],['motorola back.'],['motorola back.'],['motorola back.'],['motorola back.'],['motorola back.']},'Factor',{0.01,1,0.05,0.5,1,1,0.1,0.1,1,1,1,0.25},'Offset',{0,0,0,0,0,0,0,0,0,0,0,0},'SLDataType',{'SS_DOUBLE','SS_DOUBLE','SS_DOUBLE','SS_DOUBLE','SS_DOUBLE','SS_DOUBLE','SS_DOUBLE','SS_DOUBLE','SS_DOUBLE','SS_DOUBLE','SS_DOUBLE','SS_DOUBLE'}),'StatusSelected','no','TimeSelected','no','DeltaTimeSelected','no','BytePortSelected','no','MessageLengthSelected','no','TriggerPort',struct('Selected','no','TriggerType',0),'UserCoding',struct('Selected','no','InterfaceFile','UserDecodingFile','FcnName','UserDecodeFcn','InportSelected','no','InportWidth',1,'OutportSelected','no','OutportWidth',1),'EnablePortSelected','no','UseRXService','no','BoardType','DS1','BoardNo',2,'ControllerNo',2),'OFF',[]}},'TLCFileName',{{'rtican_rx_message','OFF',[]}})  RTISFcnParameters=struct('SFcnRTICANMessage','struct','TLCFileName','char')  RTIBlockParaDefault=struct('BoardTypeNo',4302,'BoardNo',1,'ChannelNo',1,'Parameters',struct('DataFileSupport',struct('DataFileSelectedMaster',0,'DataFileSelectedLocal',0,'DataFileName','','DataFileDate','','SelectedFile',['<no file selected>']),'Options',struct('StatusSelected',1,'TimeSelected',1,'DeltaTimeSelected',1,'BytePortSelected',0,'MessageLengthSelected',0,'TriggerPort',struct('Selected',0,'TriggerType','rising'),'UserCoding',struct('Selected',0,'InterfaceFile','UserDecodingFile','FcnName','UserDecodeFcn','InportSelected',0,'InportWidth',1,'OutportSelected',0,'OutportWidth',1),'EnablePortSelected',0,'SignalOnPortnameSelected',1,'UseRXService',0),'Message',struct('MsgOnBlocknameSelected',0,'MsgName',['RX Message'],'MsgIdFormat',0,'MsgId',100,'MsgLength',8,'NumSignals',1,'SampleTime',-1,'Signal',struct('SgnName',['RX signal'],'SgnStartBit',0,'SgnLength',8,'SgnType',0,'ModeValue',-1,'DataType',0,'SLDataType','SS_DOUBLE','ByteLayout',0,'Factor',1,'Offset',0,'Min',0,'Max',255,'SgnComment',{{}},'SgnUnit',''),'MsgIdNumFormat',0,'MsgComment',{{''}}),'Version',1.2,'general',struct('isFromLib',1)),'GroupId',struct('Group',{{'RTICAN'}},'No',1,'Behavior',{{'NAMECHANGE'}},'BlockType',{{'SINK'}},'NameChangeFlag',0),'SFcnRTICANMessage',struct('MsgType','RX','MsgName',['RX Message'],'MsgIdFormat','STD','MsgId',100,'MsgLength',8,'NumSignals',1,'SampleTime',-1,'Signal',struct('SgnName',['RX signal'],'SgnStartBit',0,'SgnLength',8,'SgnType','standard','ModeValue',-1,'DataType',['unsigned int'],'ByteLayout',['little endian'],'SLDataType','SS_DOUBLE','Factor',1,'Offset',0),'StatusSelected','yes','TimeSelected','yes','DeltaTimeSelected','yes','BytePortSelected','no','MessageLengthSelected','no','EnablePortSelected','no','UserCoding',struct('Selected','no','InterfaceFile','UserDecodingFile','FcnName','UserDecodeFcn','InportSelected','no','InportWidth',1,'OutportSelected','no','OutportWidth',1),'TriggerPort',struct('Selected','no','TriggerType','rising'),'UseRXService','no','BoardType','DS4302','BoardNo',1,'ControllerNo',1,'SFcnPortType','Scalar'),'TLCFileName','rtican_rx_message')
      settings: AttributesFormatString=Group Id: RTICAN4\n
  Out1 : Outport
  wires:
  Bus Creator/1 -> Out1/1  "Track57"
  ESR_Track57/1 -> Bus Creator/1  "CAN_TX_TRACK_RANGE_RATE_57"
  ESR_Track57/2 -> Bus Creator/2  "CAN_TX_TRACK_MED_RANGE_MODE_57"
  ESR_Track57/3 -> Bus Creator/3  "CAN_TX_TRACK_RANGE_ACCEL_57"
  ESR_Track57/4 -> Bus Creator/4  "CAN_TX_TRACK_WIDTH_57"
  ESR_Track57/5 -> Bus Creator/5  "CAN_TX_TRACK_ROLLING_COUNT_57"
  ESR_Track57/6 -> Bus Creator/6  "CAN_TX_TRACK_BRIDGE_OBJECT_57"
  ESR_Track57/7 -> Bus Creator/7  "CAN_TX_TRACK_RANGE_57"
  ESR_Track57/8 -> Bus Creator/8  "CAN_TX_TRACK_ANGLE_57"
  ESR_Track57/9 -> Bus Creator/9  "CAN_TX_TRACK_STATUS_57"
  ESR_Track57/10 -> Bus Creator/10  "CAN_TX_TRACK_ONCOMING_57"
  ESR_Track57/11 -> Bus Creator/11  "CAN_TX_TRACK_GROUPING_CHANGED_57"
  ESR_Track57/12 -> Bus Creator/12  "CAN_TX_TRACK_LAT_RATE_57"

== system Control_test/InputProcessing/RadarCanProcessing/Track58 ==
  Bus Creator : BusCreator  Inputs=12
  ESR_Track58 : rtican/RTICAN Receive (RX)   Reserved1=[]  Reserved2=[]  Reserved3=[]  Reserved4=[]  SfcnMessage=[]  Msg_Struct=[]  BoardTypeNo=[]  BoardNo=[]  ChannelNo=[]  Parameters=[]  DialogFcn=[]  UnitName=[]  Revision=[]  UnitValues=[]  DSProperties=struct('RTI',struct('Version',uint32(5),'BlockType',struct('isSLSource',uint8(1),'isSLSink',uint8(1),'isHWSource',uint8(0),'isHWSink',uint8(0),'isSetup',uint8(0),'isInline',uint8(1),'isNonInline',uint8(0),'isInterrupt',uint8(0),'isChannelwise',uint8(0)),'IOBoardType','RTICAN','UnitType','MESSAGE','Identifier','RX','DialogType','MSVC','BlockSet','RTICAN','SlaveProcessor','CAN'))  RTIBlockInterface=struct('OutputPortsWidth',int32([1 1 1 1 1 1 1 1 1 1 1 1]),'OutputPortsActive',[1 1 1 1 1 1 1 1 1 1 1 1],'OutputPortsName',{{'CAN_TX_TRACK_RANGE_RATE_58','CAN_TX_TRACK_MED_RANGE_MODE_58','CAN_TX_TRACK_RANGE_ACCEL_58','CAN_TX_TRACK_WIDTH_58','CAN_TX_TRACK_ROLLING_COUNT_58','CAN_TX_TRACK_BRIDGE_OBJECT_58','CAN_TX_TRACK_RANGE_58','CAN_TX_TRACK_ANGLE_58','CAN_TX_TRACK_STATUS_58','CAN_TX_TRACK_ONCOMING_58','CAN_TX_TRACK_GROUPING_CHANGED_58','CAN_TX_TRACK_LAT_RATE_58'}},'OutputPortsDataType',{{'SS_DOUBLE','SS_DOUBLE','SS_DOUBLE','SS_DOUBLE','SS_DOUBLE','SS_DOUBLE','SS_DOUBLE','SS_DOUBLE','SS_DOUBLE','SS_DOUBLE','SS_DOUBLE','SS_DOUBLE'}},'OutputPortsLabel',{{'CAN_TX_TRACK_RANGE_RATE_58','CAN_TX_TRACK_MED_RANGE_MODE_58','CAN_TX_TRACK_RANGE_ACCEL_58','CAN_TX_TRACK_WIDTH_58','CAN_TX_TRACK_ROLLING_COUNT_58','CAN_TX_TRACK_BRIDGE_OBJECT_58','CAN_TX_TRACK_RANGE_58','CAN_TX_TRACK_ANGLE_58','CAN_TX_TRACK_STATUS_58','CAN_TX_TRACK_ONCOMING_58','CAN_TX_TRACK_GROUPING_CHANGED_58','CAN_TX_TRACK_LAT_RATE_58'}},'OutputPortsLabelMode','ON','InputPortsWidth',int32(0),'InputPortsActive',0,'DialogFcn','rtican_message_interface_gui','BlockDisplay',{{'','center'}},'IconTransparency','on','ParameterTunableNames',{{}},'InitLevel',3,'BlockName',struct('Token',{{'ESR_Track58'}}),'SampleTime',{{0.01}},'TriggerPort',{{'none'}},'EnablePort',{{'none'}})  RTIBlockParameters=struct('BoardTypeNo',{{1,'OFF',[]}},'BoardNo',{{2,'ON',[1 16]}},'ChannelNo',{{2,'ON',[1 2]}},'Parameters',{{struct('DataFileSupport',struct('DataFileSelectedMaster',1,'DataFileSelectedLocal',0,'DataFileName','c:\users\mpc_car\documents\github\mpc-car\controller\dbcfiles\esr_dv3_64tgt.dbc|','DataFileDate',{{{['02-Nov-2012 20:32:52']},{['21-Mar-2013 13:39:53']},{['28-Sep-2011 17:08:52']}}},'SelectedFile',['<no file selected>'],'InterfaceFcn','rtican_dbc_file_parser'),'Options',struct('StatusSelected',0,'TimeSelected',0,'DeltaTimeSelected',0,'BytePortSelected',0,'MessageLengthSelected',0,'TriggerPort',struct('Selected',0,'TriggerType',0),'UserCoding',struct('Selected',0,'InterfaceFile','UserDecodingFile','FcnName','UserDecodeFcn','InportSelected',0,'InportWidth',1,'OutportSelected',0,'OutportWidth',1),'EnablePortSelected',0,'SignalOnPortnameSelected',1,'UseRXService',0),'Message',struct('MsgOnBlocknameSelected',1,'MsgName','ESR_Track58','MsgIdFormat',0,'MsgId',1337,'MsgLength',8,'NumSignals',12,'SampleTime',0.01,'Signal',struct('SgnName',{'CAN_TX_TRACK_RANGE_RATE_58','CAN_TX_TRACK_MED_RANGE_MODE_58','CAN_TX_TRACK_RANGE_ACCEL_58','CAN_TX_TRACK_WIDTH_58','CAN_TX_TRACK_ROLLING_COUNT_58','CAN_TX_TRACK_BRIDGE_OBJECT_58','CAN_TX_TRACK_RANGE_58','CAN_TX_TRACK_ANGLE_58','CAN_TX_TRACK_STATUS_58','CAN_TX_TRACK_ONCOMING_58','CAN_TX_TRACK_GROUPING_CHANGED_58','CAN_TX_TRACK_LAT_RATE_58'},'SgnStartBit',{0,14,16,26,30,31,32,43,53,56,57,58},'SgnLength',{14,2,10,4,1,1,11,10,3,1,1,6},'SgnType',{0,0,0,0,0,0,0,0,0,0,0,0},'ModeValue',{-1,-1,-1,-1,-1,-1,-1,-1,-1,-1,-1,-1},'DataType',{1,0,1,0,0,0,0,1,0,0,0,1},'ByteLayout',{2,2,2,2,2,2,2,2,2,2,2,2},'Factor',{0.01,1,0.05,0.5,1,1,0.1,0.1,1,1,1,0.25},'Offset',{0,0,0,0,0,0,0,0,0,0,0,0},'SgnComment',{{''},{''},{''},{''},{''},{''},{''},{''},{''},{''},{''},{''}},'SgnUnit',{'m/s','','m/s/s','m','','','m','deg','','','',''},'Min',{-81.92,0,-25.6,0,0,0,0,-51.2,0,0,0,-8},'Max',{81.91,3,25.55,7.5,1,0,204.7,51.1,7,0,0,7.75},'SLDataType',{'SS_DOUBLE','SS_DOUBLE','SS_DOUBLE','SS_DOUBLE','SS_DOUBLE','SS_DOUBLE','SS_DOUBLE','SS_DOUBLE','SS_DOUBLE','SS_DOUBLE','SS_DOUBLE','SS_DOUBLE'}),'MsgIdNumFormat',0,'MsgComment',{{''}}),'Version',1.2,'general',struct('isFromLib',0)),'OFF',[]}},'GroupId',{{struct('Group',{{'RTICAN'}},'No',4,'Behavior',{{'NAMECHANGE'}},'BlockType',{{'SINK'}},'NameChangeFlag',0),'OFF',[]}},'SFcnRTICANMessage',{{struct('MsgType','RX','SFcnPortType','Scalar','MsgName','ESR_Track58','MsgIdFormat','STD','MsgId',1337,'MsgLength',8,'NumSignals',12,'SampleTime',0.01,'Signal',struct('SgnName',{'CAN_TX_TRACK_RANGE_RATE_58','CAN_TX_TRACK_MED_RANGE_MODE_58','CAN_TX_TRACK_RANGE_ACCEL_58','CAN_TX_TRACK_WIDTH_58','CAN_TX_TRACK_ROLLING_COUNT_58','CAN_TX_TRACK_BRIDGE_OBJECT_58','CAN_TX_TRACK_RANGE_58','CAN_TX_TRACK_ANGLE_58','CAN_TX_TRACK_STATUS_58','CAN_TX_TRACK_ONCOMING_58','CAN_TX_TRACK_GROUPING_CHANGED_58','CAN_TX_TRACK_LAT_RATE_58'},'SgnStartBit',{0,14,16,26,30,31,32,43,53,56,57,58},'SgnLength',{14,2,10,4,1,1,11,10,3,1,1,6},'SgnType',{'standard','standard','standard','standard','standard','standard','standard','standard','standard','standard','standard','standard'},'ModeValue',{-1,-1,-1,-1,-1,-1,-1,-1,-1,-1,-1,-1},'DataType',{['signed int'],['unsigned int'],['signed int'],['unsigned int'],['unsigned int'],['unsigned int'],['unsigned int'],['signed int'],['unsigned int'],['unsigned int'],['unsigned int'],['signed int']},'ByteLayout',{['motorola back.'],['motorola back.'],['motorola back.'],['motorola back.'],['motorola back.'],['motorola back.'],['motorola back.'],['motorola back.'],['motorola back.'],['motorola back.'],['motorola back.'],['motorola back.']},'Factor',{0.01,1,0.05,0.5,1,1,0.1,0.1,1,1,1,0.25},'Offset',{0,0,0,0,0,0,0,0,0,0,0,0},'SLDataType',{'SS_DOUBLE','SS_DOUBLE','SS_DOUBLE','SS_DOUBLE','SS_DOUBLE','SS_DOUBLE','SS_DOUBLE','SS_DOUBLE','SS_DOUBLE','SS_DOUBLE','SS_DOUBLE','SS_DOUBLE'}),'StatusSelected','no','TimeSelected','no','DeltaTimeSelected','no','BytePortSelected','no','MessageLengthSelected','no','TriggerPort',struct('Selected','no','TriggerType',0),'UserCoding',struct('Selected','no','InterfaceFile','UserDecodingFile','FcnName','UserDecodeFcn','InportSelected','no','InportWidth',1,'OutportSelected','no','OutportWidth',1),'EnablePortSelected','no','UseRXService','no','BoardType','DS1','BoardNo',2,'ControllerNo',2),'OFF',[]}},'TLCFileName',{{'rtican_rx_message','OFF',[]}})  RTISFcnParameters=struct('SFcnRTICANMessage','struct','TLCFileName','char')  RTIBlockParaDefault=struct('BoardTypeNo',4302,'BoardNo',1,'ChannelNo',1,'Parameters',struct('DataFileSupport',struct('DataFileSelectedMaster',0,'DataFileSelectedLocal',0,'DataFileName','','DataFileDate','','SelectedFile',['<no file selected>']),'Options',struct('StatusSelected',1,'TimeSelected',1,'DeltaTimeSelected',1,'BytePortSelected',0,'MessageLengthSelected',0,'TriggerPort',struct('Selected',0,'TriggerType','rising'),'UserCoding',struct('Selected',0,'InterfaceFile','UserDecodingFile','FcnName','UserDecodeFcn','InportSelected',0,'InportWidth',1,'OutportSelected',0,'OutportWidth',1),'EnablePortSelected',0,'SignalOnPortnameSelected',1,'UseRXService',0),'Message',struct('MsgOnBlocknameSelected',0,'MsgName',['RX Message'],'MsgIdFormat',0,'MsgId',100,'MsgLength',8,'NumSignals',1,'SampleTime',-1,'Signal',struct('SgnName',['RX signal'],'SgnStartBit',0,'SgnLength',8,'SgnType',0,'ModeValue',-1,'DataType',0,'SLDataType','SS_DOUBLE','ByteLayout',0,'Factor',1,'Offset',0,'Min',0,'Max',255,'SgnComment',{{}},'SgnUnit',''),'MsgIdNumFormat',0,'MsgComment',{{''}}),'Version',1.2,'general',struct('isFromLib',1)),'GroupId',struct('Group',{{'RTICAN'}},'No',1,'Behavior',{{'NAMECHANGE'}},'BlockType',{{'SINK'}},'NameChangeFlag',0),'SFcnRTICANMessage',struct('MsgType','RX','MsgName',['RX Message'],'MsgIdFormat','STD','MsgId',100,'MsgLength',8,'NumSignals',1,'SampleTime',-1,'Signal',struct('SgnName',['RX signal'],'SgnStartBit',0,'SgnLength',8,'SgnType','standard','ModeValue',-1,'DataType',['unsigned int'],'ByteLayout',['little endian'],'SLDataType','SS_DOUBLE','Factor',1,'Offset',0),'StatusSelected','yes','TimeSelected','yes','DeltaTimeSelected','yes','BytePortSelected','no','MessageLengthSelected','no','EnablePortSelected','no','UserCoding',struct('Selected','no','InterfaceFile','UserDecodingFile','FcnName','UserDecodeFcn','InportSelected','no','InportWidth',1,'OutportSelected','no','OutportWidth',1),'TriggerPort',struct('Selected','no','TriggerType','rising'),'UseRXService','no','BoardType','DS4302','BoardNo',1,'ControllerNo',1,'SFcnPortType','Scalar'),'TLCFileName','rtican_rx_message')
      settings: AttributesFormatString=Group Id: RTICAN4\n
  Out1 : Outport
  wires:
  Bus Creator/1 -> Out1/1  "Track58"
  ESR_Track58/1 -> Bus Creator/1  "CAN_TX_TRACK_RANGE_RATE_58"
  ESR_Track58/2 -> Bus Creator/2  "CAN_TX_TRACK_MED_RANGE_MODE_58"
  ESR_Track58/3 -> Bus Creator/3  "CAN_TX_TRACK_RANGE_ACCEL_58"
  ESR_Track58/4 -> Bus Creator/4  "CAN_TX_TRACK_WIDTH_58"
  ESR_Track58/5 -> Bus Creator/5  "CAN_TX_TRACK_ROLLING_COUNT_58"
  ESR_Track58/6 -> Bus Creator/6  "CAN_TX_TRACK_BRIDGE_OBJECT_58"
  ESR_Track58/7 -> Bus Creator/7  "CAN_TX_TRACK_RANGE_58"
  ESR_Track58/8 -> Bus Creator/8  "CAN_TX_TRACK_ANGLE_58"
  ESR_Track58/9 -> Bus Creator/9  "CAN_TX_TRACK_STATUS_58"
  ESR_Track58/10 -> Bus Creator/10  "CAN_TX_TRACK_ONCOMING_58"
  ESR_Track58/11 -> Bus Creator/11  "CAN_TX_TRACK_GROUPING_CHANGED_58"
  ESR_Track58/12 -> Bus Creator/12  "CAN_TX_TRACK_LAT_RATE_58"
